simulink model "PIZANO_LAB5_part1_3"  (Simulink 10.0)
settings: Solver=FixedStepAuto  StartTime=0.0  StopTime=6  FixedStep=0.001  RelTol=1e-3
libraries: simulink x1
settings Model: Creator=XxaemaeThxX  LastModifiedBy=XxaemaeThxX
settings DataIOCC: SaveFormat=Dataset  ReturnWorkspaceOutputs=on
settings OptimizationCC: LifeSpan=auto
settings DebuggingCC: UnderspecifiedInitializationDetection=Simplified  MergeDetectMultiDrivingBlocksExec=error  SFUnexpectedBacktrackingDiag=error  SFNoUnconditionalDefaultTransitionDiag=error  SFExecutionAtInitializationDiag=warning  ArithmeticOperatorsInVariantConditions=error
settings HardwareCC: ProdBitPerPointer=64  ProdBitPerSizeT=64  ProdBitPerPtrDiffT=64  ProdLargestAtomicFloat=Float  ProdIntDivRoundTo=Zero  ProdEndianess=LittleEndian  ProdWordSize=64  ProdHWDeviceType=Intel->x86-64 (Windows64)
settings ModelReferenceCC: PropagateSignalLabelsOutOfModel=on
settings SFSimCC: SimUseLocalCustomCode=on  CustomCodeUndefinedFunction=FilterOut
settings RTWCC: RTWUseLocalCustomCode=on
settings CodeAppCC: StateflowObjectComments=off
settings GRTTargetCC: TargetLangStandard=C99 (ISO)  CombineOutputUpdateFcns=on  GRTInterface=off
settings ConfigComp: CovMetricSettings=dwe  CovHtmlReporting=off  CovSaveCumulativeToWorkspaceVar=off  CovSaveSingleToWorkspaceVar=off

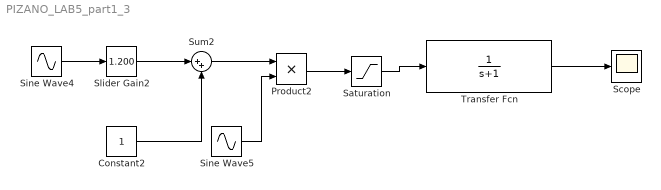
== system PIZANO_LAB5_part1_3 ==
  Constant2 : Constant
  Product2 : Product  RndMeth=Zero
  Saturation : Saturate  UpperLimit=10  LowerLimit=0
  Scope : Scope
  Sine Wave4 : Sin  Frequency=5  SampleTime=0
  Sine Wave5 : Sin  Amplitude=2  Frequency=200  SampleTime=0
  Slider Gain2 : simulink/Math Operations/Slider Gain  gain=1.200  low=0  high=2
  Sum2 : Sum  Inputs=|++
  Transfer Fcn : TransferFcn  Denominator=[1 1]
  wires:
  Transfer Fcn/1 -> Scope/1
  Saturation/1 -> Transfer Fcn/1
  Constant2/1 -> Sum2/2
  Product2/1 -> Saturation/1
  Sine Wave5/1 -> Product2/2
  Sum2/1 -> Product2/1
  Slider Gain2/1 -> Sum2/1
  Sine Wave4/1 -> Slider Gain2/1
